simulink model "SISO_MIMO_blocks_r2016b"  (R2016b)
settings: Solver=VariableStepAuto  StartTime=0.0  StopTime=10.0  RelTol=1e-3
undefined symbols (not defined in the file): freq, ScanStartTime
libraries: powerlib x8
settings Model: Creator=Yamin Sun  LastModifiedBy=Yamin Sun

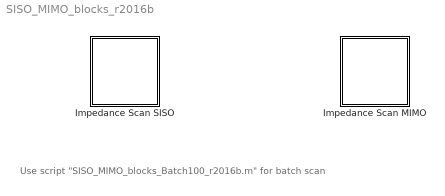
== system SISO_MIMO_blocks_r2016b ==
  note: Use script "SISO_MIMO_blocks_Batch100_r2016b.m" for batch scan
  Impedance Scan MIMO : Subsystem  mask{t_start=ScanStartTime, frequency=freq, inject_duration=1.5, record_duration=1, stable_duration=1, amp_inject=0.69e3 * 0.02, t_Ts=50e-6}
      mask prompts: t_start "Injection starting time (s)"; frequency "Frequency to be scanned (Hz)"; inject_duration "Injection durtion (s)"; record_duration "Record duration (s)"; stable_duration "Stable durtion (s)"; amp_inject "Injection magnitude. eg. 690*0.02"; t_Ts "Sample time"
      mask help:
      | |--------------Injection duration--------------|-----Stable duration------|
      |                      |-----Record duration-----|
      |
      | Record duration <= Inject duration
  Impedance Scan SISO : Subsystem  mask{t_start=ScanStartTime, frequency=freq, inject_duration=1.5, record_duration=1, stable_duration=1, amp_inject=0.69e3 * 0.02, t_Ts=50e-6}
      mask prompts: t_start "Injection starting time (s)"; frequency "Frequency to be scanned (Hz)"; inject_duration "Injection durtion (s)"; record_duration "Record duration (s)"; stable_duration "Stable durtion (s)"; amp_inject "Injection magnitude. eg. 690*0.02"; t_Ts "Sample time"
      mask help:
      | |--------------Injection duration--------------|-----Stable duration------|
      |                      |-----Record duration-----|
      |
      | Record duration <= Inject duration

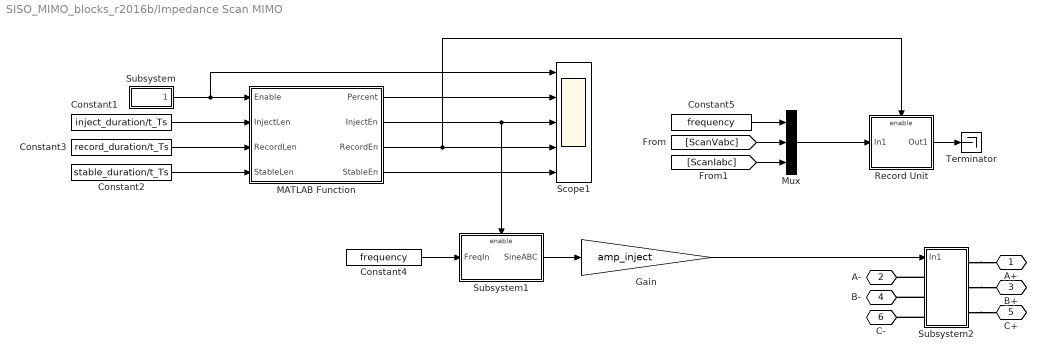
== system SISO_MIMO_blocks_r2016b/Impedance Scan MIMO ==
  Constant1 : Constant  Value=inject_duration/t_Ts
  Constant2 : Constant  Value=stable_duration/t_Ts
  Constant3 : Constant  Value=record_duration/t_Ts
  Constant4 : Constant  Value=frequency
  Constant5 : Constant  Value=frequency
  Gain : Gain  Gain=amp_inject
  MATLAB Function : MATLAB Function  TreatAsAtomicUnit=on  SystemSampleTime=t_Ts
  Mux : Mux  Inputs=3
  Record Unit : Subsystem
  Scope1 : Scope  NumInputPorts=5
  Subsystem : Subsystem  mask{t_start=t_start, t_duration=inject_duration + stable_duration}
      mask prompts: t_start "Start Time"; t_duration "Duration"
  Subsystem1 : Subsystem
  Subsystem2 : Subsystem
  Terminator : Terminator
  A+ : PMIOPort  Port=1  Side=Right
  A- : PMIOPort  Port=2  Side=Left
  B+ : PMIOPort  Port=3  Side=Right
  B- : PMIOPort  Port=4  Side=Left
  C+ : PMIOPort  Port=5  Side=Right
  C- : PMIOPort  Port=6  Side=Left
  wires:
  Mux/1 -> Record Unit/1(In1)
  Gain/1 -> Subsystem2/1(In1)
  Subsystem1/1(SineABC) -> Gain/1
  [ScanVabc] -> Mux/2
  [ScanIabc] -> Mux/3
  Record Unit/1(Out1) -> Terminator/1
  Constant4/1 -> Subsystem1/1(FreqIn)
  MATLAB Function/4(StableEn) -> Scope1/5
  MATLAB Function/3(RecordEn) -> Scope1/4, Record Unit/Enable
  MATLAB Function/2(InjectEn) -> Scope1/3, Subsystem1/Enable
  Constant5/1 -> Mux/1
  Constant3/1 -> MATLAB Function/3(RecordLen)
  Constant2/1 -> MATLAB Function/4(StableLen)
  Constant1/1 -> MATLAB Function/2(InjectLen)
  Subsystem/1(EnOut) -> MATLAB Function/1(Enable), Scope1/1
  MATLAB Function/1(Percent) -> Scope1/2
  connections:
  Subsystem2/RConn2 -- B+/RConn1
  Subsystem2/RConn1 -- A+/RConn1
  Subsystem2/LConn3 -- C-/RConn1
  Subsystem2/LConn2 -- B-/RConn1
  Subsystem2/LConn1 -- A-/RConn1
  Subsystem2/RConn3 -- C+/RConn1

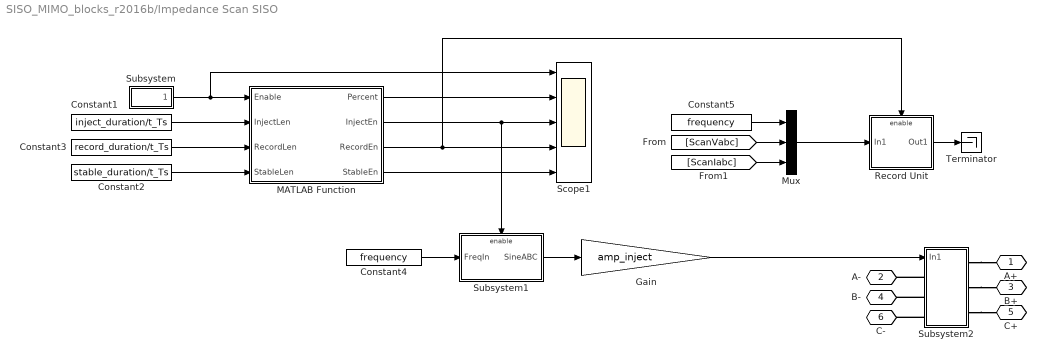
== system SISO_MIMO_blocks_r2016b/Impedance Scan SISO ==
  Constant1 : Constant  Value=inject_duration/t_Ts
  Constant2 : Constant  Value=stable_duration/t_Ts
  Constant3 : Constant  Value=record_duration/t_Ts
  Constant4 : Constant  Value=frequency
  Constant5 : Constant  Value=frequency
  Gain : Gain  Gain=amp_inject
  MATLAB Function : MATLAB Function  TreatAsAtomicUnit=on  SystemSampleTime=t_Ts
  Mux : Mux  Inputs=3
  Record Unit : Subsystem
  Scope1 : Scope  NumInputPorts=5
  Subsystem : Subsystem  mask{t_start=t_start, t_duration=inject_duration + stable_duration}
      mask prompts: t_start "Start Time"; t_duration "Duration"
  Subsystem1 : Subsystem
  Subsystem2 : Subsystem
  Terminator : Terminator
  A+ : PMIOPort  Port=1  Side=Right
  A- : PMIOPort  Port=2  Side=Left
  B+ : PMIOPort  Port=3  Side=Right
  B- : PMIOPort  Port=4  Side=Left
  C+ : PMIOPort  Port=5  Side=Right
  C- : PMIOPort  Port=6  Side=Left
  wires:
  MATLAB Function/1(Percent) -> Scope1/2
  Subsystem/1(EnOut) -> Scope1/1, MATLAB Function/1(Enable)
  Constant1/1 -> MATLAB Function/2(InjectLen)
  Constant2/1 -> MATLAB Function/4(StableLen)
  Constant3/1 -> MATLAB Function/3(RecordLen)
  Constant5/1 -> Mux/1
  MATLAB Function/2(InjectEn) -> Subsystem1/Enable, Scope1/3
  MATLAB Function/3(RecordEn) -> Record Unit/Enable, Scope1/4
  MATLAB Function/4(StableEn) -> Scope1/5
  Constant4/1 -> Subsystem1/1(FreqIn)
  Record Unit/1(Out1) -> Terminator/1
  [ScanIabc] -> Mux/3
  [ScanVabc] -> Mux/2
  Subsystem1/1(SineABC) -> Gain/1
  Gain/1 -> Subsystem2/1(In1)
  Mux/1 -> Record Unit/1(In1)
  connections:
  Subsystem2/RConn3 -- C+/RConn1
  Subsystem2/LConn1 -- A-/RConn1
  Subsystem2/LConn2 -- B-/RConn1
  Subsystem2/LConn3 -- C-/RConn1
  Subsystem2/RConn1 -- A+/RConn1
  Subsystem2/RConn2 -- B+/RConn1

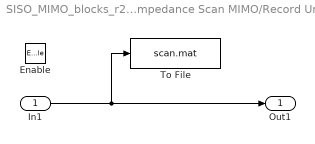
== system SISO_MIMO_blocks_r2016b/Impedance Scan MIMO/Record Unit ==
  In1 : Inport
  Enable : EnablePort
  To File : ToFile  Filename=scan.mat  MatrixName=scan  SampleTime=t_Ts
  Out1 : Outport
  wires:
  In1/1 -> Out1/1, To File/1

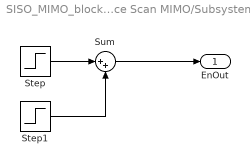
== system SISO_MIMO_blocks_r2016b/Impedance Scan MIMO/Subsystem ==
  Step : Step  Time=t_start  SampleTime=t_Ts
  Step1 : Step  Time=t_start+t_duration  After=-1  SampleTime=t_Ts
  Sum : Sum  Inputs=|++
  EnOut : Outport
  wires:
  Sum/1 -> EnOut/1
  Step/1 -> Sum/1
  Step1/1 -> Sum/2

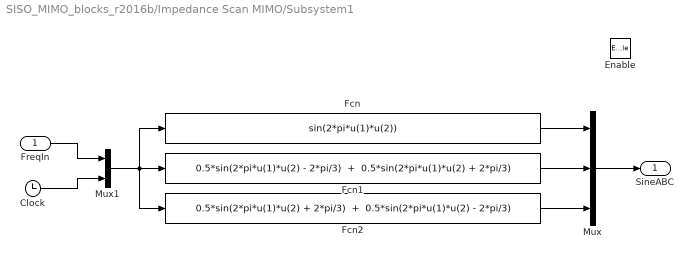
== system SISO_MIMO_blocks_r2016b/Impedance Scan MIMO/Subsystem1 ==
  FreqIn : Inport
  Enable : EnablePort
  Clock : Clock
  Fcn : Fcn  Expr=sin(2*pi*u(1)*u(2))
  Fcn1 : Fcn  Expr="0.5*sin(2*pi*u(1)*u(2) - 2*pi/3)  +  0.5*sin(2*pi*u(1)*u(2) + 2*pi/3)"
  Fcn2 : Fcn  Expr="0.5*sin(2*pi*u(1)*u(2) + 2*pi/3)  +  0.5*sin(2*pi*u(1)*u(2) - 2*pi/3)"
  Mux : Mux  Inputs=3
  Mux1 : Mux  Inputs=2
  SineABC : Outport
  wires:
  Fcn1/1 -> Mux/2
  Fcn/1 -> Mux/1
  Fcn2/1 -> Mux/3
  Mux/1 -> SineABC/1
  Mux1/1 -> Fcn2/1, Fcn/1, Fcn1/1
  FreqIn/1 -> Mux1/1
  Clock/1 -> Mux1/2

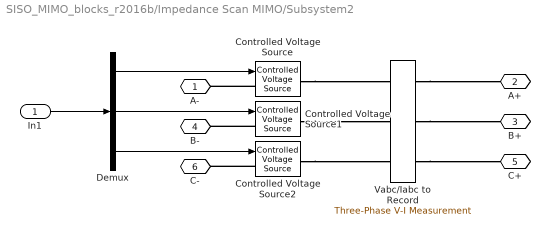
== system SISO_MIMO_blocks_r2016b/Impedance Scan MIMO/Subsystem2 ==
  In1 : Inport
  Controlled Voltage Source : powerlib/Electrical Sources/Controlled Voltage Source  Initialize=on  Source_Type=AC  Amplitude=0  Phase=0  Frequency=0  Measurements=None
  Controlled Voltage Source1 : powerlib/Electrical Sources/Controlled Voltage Source  Initialize=on  Source_Type=AC  Amplitude=0  Phase=0  Frequency=0  Measurements=None
  Controlled Voltage Source2 : powerlib/Electrical Sources/Controlled Voltage Source  Initialize=on  Source_Type=AC  Amplitude=0  Phase=0  Frequency=0  Measurements=None
  Demux : Demux  Outputs=3
  Vabc/Iabc to Record : powerlib/Measurements/Three-Phase V-I Measurement  VoltageMeasurement=phase-to-ground  SetLabelV=on  LabelV=ScanVabc  Vpu=off  VpuLL=off  CurrentMeasurement=yes  SetLabelI=on  LabelI=ScanIabc  Ipu=off  Pbase=100e6  Vbase=500e3  OutputType=Complex  PhasorSimulation=off  PSBequivalent=0
  A- : PMIOPort  Port=1  Side=Left
  A+ : PMIOPort  Port=2  Side=Right
  B+ : PMIOPort  Port=3  Side=Right
  B- : PMIOPort  Port=4  Side=Left
  C+ : PMIOPort  Port=5  Side=Right
  C- : PMIOPort  Port=6  Side=Left
  wires:
  Demux/3 -> Controlled Voltage Source2/1
  Demux/2 -> Controlled Voltage Source1/1
  Demux/1 -> Controlled Voltage Source/1
  In1/1 -> Demux/1
  connections:
  Vabc/Iabc to Record/RConn1 -- A+/RConn1
  Controlled Voltage Source/RConn1 -- Vabc/Iabc to Record/LConn1
  Controlled Voltage Source1/RConn1 -- Vabc/Iabc to Record/LConn2
  Controlled Voltage Source2/RConn1 -- Vabc/Iabc to Record/LConn3
  Vabc/Iabc to Record/RConn3 -- C+/RConn1
  Controlled Voltage Source/LConn1 -- A-/RConn1
  Controlled Voltage Source1/LConn1 -- B-/RConn1
  Vabc/Iabc to Record/RConn2 -- B+/RConn1
  Controlled Voltage Source2/LConn1 -- C-/RConn1

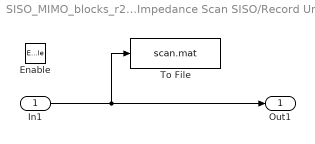
== system SISO_MIMO_blocks_r2016b/Impedance Scan SISO/Record Unit ==
  In1 : Inport
  Enable : EnablePort
  To File : ToFile  Filename=scan.mat  MatrixName=scan  SampleTime=t_Ts
  Out1 : Outport
  wires:
  In1/1 -> To File/1, Out1/1

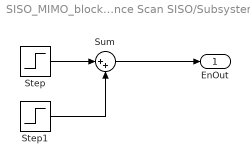
== system SISO_MIMO_blocks_r2016b/Impedance Scan SISO/Subsystem ==
  Step : Step  Time=t_start  SampleTime=t_Ts
  Step1 : Step  Time=t_start+t_duration  After=-1  SampleTime=t_Ts
  Sum : Sum  Inputs=|++
  EnOut : Outport
  wires:
  Step1/1 -> Sum/2
  Step/1 -> Sum/1
  Sum/1 -> EnOut/1

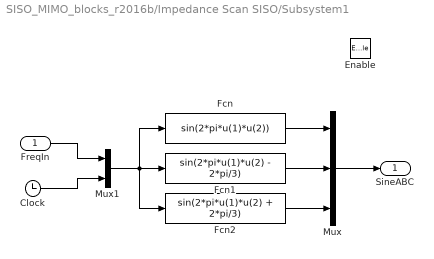
== system SISO_MIMO_blocks_r2016b/Impedance Scan SISO/Subsystem1 ==
  FreqIn : Inport
  Enable : EnablePort
  Clock : Clock
  Fcn : Fcn  Expr=sin(2*pi*u(1)*u(2))
  Fcn1 : Fcn  Expr=sin(2*pi*u(1)*u(2) - 2*pi/3)
  Fcn2 : Fcn  Expr=sin(2*pi*u(1)*u(2) + 2*pi/3)
  Mux : Mux  Inputs=3
  Mux1 : Mux  Inputs=2
  SineABC : Outport
  wires:
  Clock/1 -> Mux1/2
  FreqIn/1 -> Mux1/1
  Mux1/1 -> Fcn1/1, Fcn/1, Fcn2/1
  Mux/1 -> SineABC/1
  Fcn2/1 -> Mux/3
  Fcn/1 -> Mux/1
  Fcn1/1 -> Mux/2

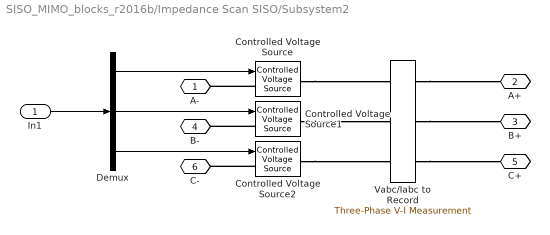
== system SISO_MIMO_blocks_r2016b/Impedance Scan SISO/Subsystem2 ==
  In1 : Inport
  Controlled Voltage Source : powerlib/Electrical Sources/Controlled Voltage Source  Initialize=on  Source_Type=AC  Amplitude=0  Phase=0  Frequency=0  Measurements=None
  Controlled Voltage Source1 : powerlib/Electrical Sources/Controlled Voltage Source  Initialize=on  Source_Type=AC  Amplitude=0  Phase=0  Frequency=0  Measurements=None
  Controlled Voltage Source2 : powerlib/Electrical Sources/Controlled Voltage Source  Initialize=on  Source_Type=AC  Amplitude=0  Phase=0  Frequency=0  Measurements=None
  Demux : Demux  Outputs=3
  Vabc/Iabc to Record : powerlib/Measurements/Three-Phase V-I Measurement  VoltageMeasurement=phase-to-ground  SetLabelV=on  LabelV=ScanVabc  Vpu=off  VpuLL=off  CurrentMeasurement=yes  SetLabelI=on  LabelI=ScanIabc  Ipu=off  Pbase=100e6  Vbase=500e3  OutputType=Complex  PhasorSimulation=off  PSBequivalent=0
  A- : PMIOPort  Port=1  Side=Left
  A+ : PMIOPort  Port=2  Side=Right
  B+ : PMIOPort  Port=3  Side=Right
  B- : PMIOPort  Port=4  Side=Left
  C+ : PMIOPort  Port=5  Side=Right
  C- : PMIOPort  Port=6  Side=Left
  wires:
  In1/1 -> Demux/1
  Demux/1 -> Controlled Voltage Source/1
  Demux/2 -> Controlled Voltage Source1/1
  Demux/3 -> Controlled Voltage Source2/1
  connections:
  Controlled Voltage Source2/LConn1 -- C-/RConn1
  Vabc/Iabc to Record/RConn2 -- B+/RConn1
  Controlled Voltage Source1/LConn1 -- B-/RConn1
  Controlled Voltage Source/LConn1 -- A-/RConn1
  Vabc/Iabc to Record/RConn3 -- C+/RConn1
  Controlled Voltage Source2/RConn1 -- Vabc/Iabc to Record/LConn3
  Controlled Voltage Source1/RConn1 -- Vabc/Iabc to Record/LConn2
  Controlled Voltage Source/RConn1 -- Vabc/Iabc to Record/LConn1
  Vabc/Iabc to Record/RConn1 -- A+/RConn1

== matlab function SISO_MIMO_blocks_r2016b/Impedance Scan MIMO/MATLAB Function ==
  data: Percent output; Enable input; InjectLen input; RecordLen input; StableLen input; InjectEn output; RecordEn output; StableEn output
function [Percent, InjectEn, RecordEn, StableEn] = fcn(Enable, InjectLen, RecordLen, StableLen)

persistent cnt_idx;
if isempty(cnt_idx)
    cnt_idx = 0;
    InjectEn = 0;
    RecordEn = 0;
    StableEn = 0;
else
    if Enable == 1
        if cnt_idx > 0 && cnt_idx <= (InjectLen-RecordLen)
            InjectEn = 1;
            RecordEn = 0;
            StableEn = 0;
        elseif cnt_idx > (InjectLen-RecordLen) && cnt_idx <= InjectLen
            InjectEn = 1;
            RecordEn = 1;
            StableEn = 0;
        elseif cnt_idx > InjectLen && cnt_idx <= (InjectLen + StableLen)
            InjectEn = 0;
            RecordEn = 0;
            StableEn = 1;
        else
            InjectEn = 0;
            RecordEn = 0;
            StableEn = 0;
        end
        cnt_idx = cnt_idx + 1;
    else
        cnt_idx = 0;
        InjectEn = 0;
        RecordEn = 0;
        StableEn = 0;
    end
end

Percent = cnt_idx;

== matlab function SISO_MIMO_blocks_r2016b/Impedance Scan SISO/MATLAB Function ==
  data: Percent output; Enable input; InjectLen input; RecordLen input; StableLen input; InjectEn output; RecordEn output; StableEn output
function [Percent, InjectEn, RecordEn, StableEn] = fcn(Enable, InjectLen, RecordLen, StableLen)

persistent cnt_idx;
if isempty(cnt_idx)
    cnt_idx = 0;
    InjectEn = 0;
    RecordEn = 0;
    StableEn = 0;
else
    if Enable == 1
        if cnt_idx > 0 && cnt_idx <= (InjectLen-RecordLen)
            InjectEn = 1;
            RecordEn = 0;
            StableEn = 0;
        elseif cnt_idx > (InjectLen-RecordLen) && cnt_idx <= InjectLen
            InjectEn = 1;
            RecordEn = 1;
            StableEn = 0;
        elseif cnt_idx > InjectLen && cnt_idx <= (InjectLen + StableLen)
            InjectEn = 0;
            RecordEn = 0;
            StableEn = 1;
        else
            InjectEn = 0;
            RecordEn = 0;
            StableEn = 0;
        end
        cnt_idx = cnt_idx + 1;
    else
        cnt_idx = 0;
        InjectEn = 0;
        RecordEn = 0;
        StableEn = 0;
    end
end

Percent = cnt_idx;
